simulink model "TrailerSoftware"  (R2019b)
settings: Solver=FixedStepDiscrete  StartTime=0.0  StopTime=inf  FixedStep=update  RelTol=1e-3  EnableMultiTasking=on
values from neighbouring files (symbols this model uses):
  countmax1 = 2500    [ProductionMfile.m]
  countmax2 = 2500    [ProductionMfile.m]
  HeaterIntGain = .0008    (= 0.0008)    [ProductionMfile.m]
  HeatGain = 10    [ProductionMfile.m]
  Intll = 0    [ProductionMfile.m]
  MaxCondPressure = 350    [ProductionMfile.m]
  MinSP = 1    [ProductionMfile.m]
  PostGain100 = 0.0002    [ProductionMfile.m]
  PostGain150 = 0.0005    [ProductionMfile.m]
  PostGain200 = 0.0004    [ProductionMfile.m]
  PostGain300 = 0.0008    [ProductionMfile.m]
  PostInit150 = 12    [ProductionMfile.m]
  PostIntulC = 65    [ProductionMfile.m]
  PostPGain = 0    [ProductionMfile.m]
  PreGain100 = 0.0005    [ProductionMfile.m]
  PreGain150 = 0.0005    [ProductionMfile.m]
  PreGain200 = 0.0003    [ProductionMfile.m]
  PreGain300 = 0.0008    [ProductionMfile.m]
  PreInit150 = 30    [ProductionMfile.m]
  PreIntulC = 65    [ProductionMfile.m]
  PreIntulDH = 65    [ProductionMfile.m]
  PrePGain = 0    [ProductionMfile.m]
  SatPress = [10 20 30 40 50 60 70 80 90 100 110 120 130 140 150 160 170      180 190 200 210 220 230 240 250 260 270 280 290 300 310 320 330      340 350 360 370 380 390 400 410 420 430 440 450 460 470 480 490      500]    [ProductionMfile.m]
  SatTemp = [-29.497 -2.4046 15.401 29.047 40.267 49.88 58.338 65.922 72.819      79.159 85.037 90.526 95.68 100.55 105.16 109.54 113.73 117.73 121.57      125.26 128.82 132.25 135.56 138.77 141.88 144.89 147.82 150.67 153.44      156.15 158.78 161.35 163.85 166.3 168.7 171.04 173.33 175.58 177.77      179.93 182.04 184.11 186.14 188.14 190.09 192.01 193.9 195.75 197.58      199.37]    [ProductionMfile.m]
  SHGain = 2    [ProductionMfile.m]
  SizeCANMatrix = 80    [ProductionMfile.m]
  SizeCOBIDVector = 10    [ProductionMfile.m]
  update = 0.002    [ProductionMfile.m]
undefined symbols (not defined in the file or in its folder): DiscIntNeverNeededParam, PostDGain, PreDGain, Ratio100, Ratio150, Ratio200, Ratio300
libraries: simulink x60, c2837xDlib x35, xpcutilitieslib x24, c2802xlib x8, c280xlib x7, etargetslib x4, svdutilitieslib x2, c2000lib x1
(part 6 of 8)

== matlab function TrailerSoftware/Subsystem/State Machine ==
  data: OutputDiscretes1Out output double size=[16,1]; modeout output; powerselectout output; OpenByPassValve output; DiscreteInput1 input; time input; MBV input; OutputDiscretes2Out output double size=[16,1]; DiscreteInput2 input; MaxPressureout output; ReadATMPress output; CR3 input; CR4 input; FRSettingOut output; stateout output; StartAC output; SuctionPressure input; CurrentStateOut output; StartACDH output; HeaterTempCom output; UseHeater output; CoolTempCom output; BiPassExpanValveCom output; CompressorOnOut output; ResetAC output; CompExitTemp input; warning1 output; warning2 output; warning3 output; fault1 output; fault2 output; fault3 output; debugout output; CR3out output; CR4out output; CompLiquidLevel2High input; MaxCondPressure parameter; CompHeaterTemp input; MinSP parameter; LiquidInjectionOnOut output; DuctTemp input; PressureFB input; Patm input; PreFreezeWarn input; ResetSM output; InitSM output; TempPot input; ByPassValvePos input; FacilityVoltage input; CondenserPressure input; BlowerLevel input; GearBoxLevel input; Latch output; estopout output; Initcomplete1 input; Initcomplete2 input; td input; GearboxTempSwitch input; PrePlusPost input
function [OutputDiscretes1Out,modeout,powerselectout,OpenByPassValve,...
    OutputDiscretes2Out,MaxPressureout,ReadATMPress,FRSettingOut,stateout,...
    StartAC,CurrentStateOut,StartACDH,HeaterTempCom,...
    UseHeater,CoolTempCom,BiPassExpanValveCom,CompressorOnOut,...
    ResetAC,warning1,warning2,warning3,fault1,fault2,fault3,debugout,...
    CR3out,CR4out,LiquidInjectionOnOut,ResetSM,InitSM,Latch,estopout]...
       = fcn(DiscreteInput1,time,MBV,DiscreteInput2,CR3,CR4,...
    SuctionPressure,CompExitTemp,CompLiquidLevel2High,MaxCondPressure,...
    CompHeaterTemp,MinSP,DuctTemp,PressureFB,Patm,PreFreezeWarn,...
    TempPot,ByPassValvePos,FacilityVoltage,...
    CondenserPressure,BlowerLevel,GearBoxLevel,...
    Initcomplete1,Initcomplete2,td,GearboxTempSwitch,PrePlusPost)
persistent  state tmode UseGenerator UseFacility CompressorHeaterOn...
    time1 time2 Motor powerselect ACShutoffOn EngineOn...
    Fault Latch1 Latch3 Latch4 Latch5 Latch6 Latch7 Latch8...
    Latch9 Latch10 Latch11 Latch12 Latch13 time4 nextstate debug oldtmode...   
    FRSetting MaxPressure Fan1On Fan2On FaultLightOn Latch2...
    CurrentState Warning BypassACShutdown DynagenFault Overpressure...
    Latch14 Latch15 LiquidInjectionOn WarningLightOn CompressorOn Idle ...
    Fan1Onlatch Fan1Ontime Fan2Onlatch Fan2Ontime MotorOnlatch ...
    MotorOntime CompressorOnlatch CompressorOntime HGBypass OilOntime ...
    Oillatch LatchMinSP timerMinSP latchComp OverPressureLatch ...
    timeoverpress Latch16 time5 time6 time7 time8 Latch18 OilPumpOn
    
%Only Comments added 2020/01/11
if isempty(Latch1)
    Latch1 = 0;
    Latch2 = 1;
    Latch3 = 0;
    Latch4 = 0;
    Latch5 = 0;
    Latch6 = 0;
    Latch7 = 0;
    Latch8 = 0;
    Latch9 = 0;
    Latch10 = 0;
    Latch11 = 0;
    Latch12 = 0;
    Latch13 = 0;
    Latch14 = 0;
    Latch15 = 0;
    Latch18 = 0;
    time1 = time;
    time2 = time;
    time4 = time;
    state = 0;
    tmode = 0;
    powerselect = 0;
    FRSetting = 0;
    MaxPressure = 1;
    Fault = zeros(41,1);
    CurrentState = 0;
    Warning = zeros(20,1);
    BypassACShutdown = 0;
    DynagenFault = 0;
    nextstate = 0;
    debug = 0;
    oldtmode = 0;
    Overpressure = 2;
    LiquidInjectionOn = 0;
    Motor = 0;
    ACShutoffOn = 0;
    HGBypass = 0;
    UseGenerator = 0;
    UseFacility = 0;
    CompressorHeaterOn = 0;
    EngineOn = 0;
    Fan1On = 0;
    Fan2On = 0;
    FaultLightOn = 0;
    WarningLightOn = 0;
    CompressorOn = 0;
    Idle = 0;
    Fan1Onlatch = 0;
    Fan1Ontime = 0;
    Fan2Onlatch = 0;
    Fan2Ontime = 0;
    MotorOnlatch = 0;
    MotorOntime = 0;
    CompressorOnlatch = 0;
    CompressorOntime = 0;
    OilPumpOn = 0;
    OilOntime = time;
    Oillatch = 0;
    LatchMinSP = 0;
    timerMinSP = 0;
    latchComp = 0;
    OverPressureLatch = 0;
    timeoverpress = 0;
    CompLiquidLevelLatch = 0;
    Latch16 = 0;
    time5 = 0;
    time6 = 0;
    time7 = 0;
    time8 = 0;
end

% Modbus Vector
% MBV(1,1) = SystemStateValue;
% MBV(2,1) = RunningStateValue;
% MBV(3,1) = EventBitMap1ValueA;
% MBV(4,1) = EventBitMap1ValueB;
% MBV(5,1) = EventBitMap2ValueA;
% MBV(6,1) = EventBitMap2ValueB;
% MBV(7,1) = FaultBitMapValueA;
% MBV(8,1) = FaultBitMapValueA;
% MBV(9,1) = WarningBitMapValueA;
% MBV(10,1) = WarningBitMapValueB;
% MBV(11,1) = GenFreqValue;
% MBV(12,1) = GenVoltValueA;
% MBV(13,1) = GenVoltValueB;
% MBV(14,1) = GenVoltValueC;
% MBV(15,1) = GenCurValueA;
% MBV(16,1) = GenCurValueB;
% MBV(17,1) = GenCurValueC;
% MBV(18,1) = EngineTempValue;
% MBV(19,1) = EngineOilPressValue;
% MBV(20,1) = FuelLevelValue;
% MBV(21,1) = BatteryVoltValue;
% MBV(22,1) = EngineRunHoursValue;

% Board 1
% DisIn1
% 1) Transmission Switch #1
% 2) Transmission Switch #2
% 3) Transmission Switch #3
% 4) Transmission Switch #4  (Input 4 No Longer Used, Trans Switch4 is now
%                             Input 16)
% 5) Blower Motor Over Heat
% 6) spare
% 7) Stop
% 8) spare
% 9) System Mode Switch Position 1
% 10) System Mode Switch Position 2
% 11) System Mode Switch Position 3
% 12) System Mode Switch Position 4
% 13)  Blower #2 Temp Switch            Power Mode Switch NO 
% 14) Blower #1 Temp Switch             Power Mode Switch NC
% 15) Reset/Start
% 16) Blower #3 Temp Switch   (Now Transmission Switch 4 2019/11/13)


% Discrete Output 1 - hot gas bypass
% Discrete Output 2 - Compressor #3 valve
% Discrete Output 3 - Compressor liquid injection
% Discrete Output 4 - Warning light
% Discrete Output 5 - Fault light
% Discrete Output 6 - A/C shutoff valve
% Discrete Output 7 - Compressor #4 valve
% Discrete Output 8 - Pre dir 
% Discrete Output 9 - Pre step
% Discrete Output 10 - Post dir
% Discrete Output 11 - Spare
% Discrete Output 12 - Spare
% Discrete Output 13 - Spare
% Discrete Output 14 - Spare
% Discrete Output 15 - Spare
% Discrete Output 16 - Spare
% A/D
% ScaledAtoD1 1 -  
% ScaledAtoD1 2 -  
% ScaledAtoD1 3 -  
% ScaledAtoD1 4 -  
% ScaledAtoD1 5 -  
% ScaledAtoD1 6 -  
% ScaledAtoD1 7 - 
% ScaledAtoD1 8 -  
% CAN A/D


% Board 2
% Discrete Input 1 - Fan 1 current switch
% Discrete Input 2 - Operatetor Shutdown
% Discrete Input 3 - Water pump current switch
% Discrete Input 4 - Fan 2 current switch
% Discrete Input 5 - Estop
% Discrete Input 6 - Oil pump current switch
% Discrete Input 7 - Facility current switch
% Discrete Input 8 - Timer relay
% Discrete Input 9 - Motor current switch
% Discrete Input 10 - Generator current switch
% Discrete Input 11 - spare
% Discrete Input 12 - Compressor 1 current switch
% Discrete Input 13 - spare
% Discrete Input 14 - spare
% Discrete Input 15 - Compressor 2 current switch
% Discrete Input 16 - spare

% Discrete 1 Output - Spare
% Discrete 2 Output - Idle
% Discrete 3 Output - Oil Pump Relay
% Discrete 4 Output - Compressor Contactor 1
% Discrete 5 Output - Compressor Contactor 2
% Discrete 6 Output - Spare
% Discrete 7 Output - Fan1
% Discrete 8 Output - Fan2
% Discrete 9 Output - Genset
% Discrete 10 Output - Facility
% Discrete 11 Output - Spare
% Discrete 12 Output - Engine On/Off
% Discrete 13 Output - Compressor Heater
% Discrete 14 Output - Spare
% Discrete 15 Output - Water Pump
% Discrete 16 Output - Motor
estopout = 0;
Latch = uint32(0);
Latch = bitset(Latch,1,uint8(Latch1));
Latch = bitset(Latch,2,uint8(Latch2));
Latch = bitset(Latch,3,uint8(Latch3));
Latch = bitset(Latch,4,uint8(Latch4));
Latch = bitset(Latch,5,uint8(Latch5));
Latch = bitset(Latch,6,uint8(Latch6));
Latch = bitset(Latch,7,uint8(Latch7));
Latch = bitset(Latch,8,uint8(Latch8));
Latch = bitset(Latch,9,uint8(Latch9));
Latch = bitset(Latch,10,uint8(Latch10));
Latch = bitset(Latch,11,uint8(Latch11));
Latch = bitset(Latch,12,uint8(Latch12));
Latch = bitset(Latch,13,uint8(Latch13));
Latch = bitset(Latch,14,uint8(Latch14));
Latch = bitset(Latch,15,uint8(Latch15));

OutputDiscretes1Out = zeros(16,1);
OutputDiscretes2Out = zeros(16,1);
OpenByPassValve = 0;
MaxPressureout = MaxPressure;
ReadATMPress = 0;
FRSettingOut = FRSetting;
stateout = state;
countwarning = 0;
warning1 = 0;
warning2 = 0;
warning3 = 0;
Reset = DiscreteInput1(15,1);
StartAC = 0;
CurrentStateOut = CurrentState;
StartACDH = 0;
UseHeater = 0;
BiPassExpanValveCom = 0;
CR3BP = CR3;
CR4BP = CR4;
Estop = DiscreteInput2(5); % Estop = 1 OK
if time < 5 
    modeout = 0;
    powerselectout = 0;
    debugout = 0;
    HeaterTempCom = 0;
    CoolTempCom = 0;
    CompressorOnOut = 0;
    ResetAC = 0;
    fault1 = 0;
    fault2 = 0;
    fault3 = 0;
    CR3out = 0;
    CR4out = 0;
    LiquidInjectionOnOut = 0;
    ResetSM = 1;
    InitSM = 0;
    ReadATMPress = 1; 
    return
end
ResetAC = 1;
ResetSM = 0;
InitSM = 0;
if time > 5 && Initcomplete1 == 0 && Initcomplete2 == 0
    InitSM = 1;
end
OvertempVector = zeros(4,1);
if DiscreteInput1(14) == 0  % Blower #1
    OvertempVector(1,1) = 1;
end
if DiscreteInput1(13) == 0 % Blower #2
    OvertempVector(2,1) = 1;
end
% Blower3 temp input now used for transmission switch 4, 2019-11-13
%if DiscreteInput1(16) == 0 % Blower #3
%    OvertempVector(3,1) = 1;
%end 
if GearboxTempSwitch == 0
    OvertempVector(4,1) = 1;
end
SysModePos1 = DiscreteInput1(8);
SysModePos2 = DiscreteInput1(9);
SysModePos3 = DiscreteInput1(6);
SysModePos4 = DiscreteInput1(7);
PowerModeNO = DiscreteInput1(11);
PowerModeNC = DiscreteInput1(10);
Stop = DiscreteInput1(12);
Fan1CurrentSwitch = DiscreteInput2(1);
Fan2CurrentSwitch = DiscreteInput2(4);
OilPumpCurrentSwitch = DiscreteInput2(6);
Timer = DiscreteInput2(8);
MotorIsOn = DiscreteInput2(9);
Compressor1CurrentSwitch = DiscreteInput2(12);
Compressor2CurrentSwitch = DiscreteInput2(15);
MotorNotOverheat = 1;
CompressorShutDown = DiscreteInput2(8,1);
LimitSwitch1 = DiscreteInput1(1);
LimitSwitch2 = DiscreteInput1(2);
LimitSwitch3 = DiscreteInput1(3);
LimitSwitch4 = DiscreteInput1(16);
% Blower3 temp input, DiscreteInput1(16), now used for
% transmission limit switch4, instead of DiscreteInput1(4), 2019-11-13
 BlowerOilFault = 0;
if BlowerLevel >= 1.4
    BlowerOilFault = 1;
end
 GearBoxOilFault = 0;
%if GearBoxLevel >= 1.4
%    GearBoxOilFault = 1;
%end
CompLiquidLevelFault = 0;
if (CompLiquidLevel2High < 1.4) 
    if Latch16 == 0
        time5 = time;
        Latch16 = 1;
    end
    if (time - time5) > 30
        CompLiquidLevelFault = 1;
    end
else
    Latch16 = 0;
end
% Determine the selection of the power switch
if PowerModeNO == 0 && PowerModeNC == 0 % Off
    powerselect = 0; % 
end
if  PowerModeNO == 1 && PowerModeNC == 0
    powerselect = 1; % Generator
end
if PowerModeNO == 1 && PowerModeNC == 1
    powerselect = 2; % Facilility Power
end
% Determine the selction of the mode switch
% Idle = Discrete Input 8 is 1
% De-Hum = Discrete Input 11 is 1
% Cool = Discrete Input 9 is 1
% Heat = Discrete Input 10 is 1
if SysModePos1 == 1
    tmode = 1; % Idle
end
if SysModePos2 == 1
    tmode = 2; % De-Hum
end
if SysModePos3 == 1
    tmode = 3; % Cool
end   
if SysModePos4 == 1
    tmode = 4; % Heat Blower
end 
if Reset == 1 && Latch8 == 1 && Latch10 == 0 % Reset is pushed
    Latch3 = 1;
    oldtmode = tmode;
    Latch10 = 1;
end
% Determine the blower set point
if LimitSwitch1 == 1 && LimitSwitch2 == 0 ... % 100 lbm/min
        && LimitSwitch3 == 0 && LimitSwitch4 == 1  
    FRSetting = 100;
    MaxPressure = 5.75;
    Overpressure = 6.5;
end
if LimitSwitch1 == 1 && LimitSwitch2 == 0 ...  % 150 lbm/min
        && LimitSwitch3 == 1 && LimitSwitch4 == 0 
    FRSetting = 150;
    MaxPressure = 5.75;
    Overpressure = 6.5;
end
if LimitSwitch1 == 0 && LimitSwitch2 == 1 ... % 200 lbm/min
        && LimitSwitch3 == 0 && LimitSwitch4 == 1  
    FRSetting = 200;
    MaxPressure = 3.25;
    Overpressure = 4.25;
end
if LimitSwitch1 == 0 && LimitSwitch2 == 1 ... % 300 lbm/min
        && LimitSwitch3 == 1 && LimitSwitch4 == 0  
    FRSetting = 300;
    MaxPressure = 1.25;
    Overpressure = 3.00;
end 

%Transitions from one mode to another
if Reset == 1 && (CurrentState == 700 || CurrentState == 1300 || ...
        CurrentState == 2300 || CurrentState == 3300 || CurrentState == 4300 ||...
        CurrentState ==5300 || CurrentState == 6300 || ...
        CurrentState == 700 || CurrentState == 700) && tmode ~= oldtmode     
   if powerselect == 1 && tmode == 1 && oldtmode == 3  % Generator from Cool to idle
       BypassACShutdown = 0;
       state = 700;
       time1 = time;
   end
   if powerselect == 1 && tmode == 1 && oldtmode == 2  % Generator from Dehumidifying to idle
       BypassACShutdown = 0;
       state = 700;
       time1 = time;
   end
   if powerselect == 1 && tmode == 1 && oldtmode == 4  % Generator from Blower and Heat to idle
       BypassACShutdown = 1;
       state = 700;
       time1 = time;
   end
   if powerselect == 1 && tmode == 2 && oldtmode == 1  % From Idle to De-Hum
        state = 1100;
        time1 = time;
    end
   if powerselect == 1 && tmode == 3 && oldtmode == 1  % Generator from idle to Cool
       state = 2100;
       time1 = time;
   end
   if powerselect == 1 && tmode == 4 && oldtmode == 1  % Generator from idle to Blower and Heat
       state = 3100;
       time1 = time;
   end
   if powerselect == 1 && tmode == 2 && oldtmode == 3 % Generator and Cool to Generator and Dehumidifying
       state = 1300;
       time1 = time;
   end
   if powerselect == 1 && tmode == 3 && oldtmode == 2  % Generator and Dehumidifying to Generator and Cool
       state = 2100;
       time1 = time;
   end
   if powerselect == 1 && tmode == 4 && oldtmode == 2  % Generator Power and Dehumidifying to Generator Power and Heat
       state = 1400;
       time1 = time;
   end
   if powerselect == 1 && tmode == 4 && oldtmode == 3  % Generator and Cool to Generator Heat
       state = 2400;
       time1 = time;
   end
   if powerselect == 1 && tmode == 3 && oldtmode == 4   % Generator Heat to Generator and Cool
       state = 2220;
       time1 = time;
   end
   if powerselect == 1 && tmode == 2 && oldtmode == 4   % Generator Heat to Generator and Dehumidify
       state = 1220;
       time1 = time;
   end
   if powerselect == 2 && tmode == 2 && oldtmode == 2  % Facilility Power and Cool to Facilility Power and Dehumidifying
       state = 4300;
       time1 = time;
   end
   if powerselect == 2 && tmode == 3 && oldtmode == 2  % Facilility Power and Dehumidifying to Facilility Power and Cool
       state = 5300;
       time1 = time;
   end
   if powerselect == 2 && tmode == 3 && oldtmode == 1  % Facilility Power and Dehumidifying to Facilility Power and Heat
       state = 4400;
       time1 = time;
   end
   if powerselect == 2 && tmode == 4 && oldtmode == 3  % Facilility Power and Cool to Facilility Power Heat
       state = 5400;
       time1 = time;
   end
   if powerselect == 2 && tmode == 3 && oldtmode == 4   % Facilility Power Heat to Facilility Power and Cool
       state = 5220;
       time1 = time;
   end
   if powerselect == 2 && tmode == 2 && oldtmode == 4   % Facilility Power Heat to Facilility Power and Cool
       state = 4220;
       time1 = time;
   end    
   oldtmode = tmode;
end
    
if Latch11 == 0 % Used to set initial configuration
    if tmode == 1 &&  powerselect == 0 && Latch9 == 0 
        Latch8 = 1;  % Latch8 indicates that the powerselect and tmode have been set to 0
        Latch3 = 0;  % Latch3 indicates that the reset button has been pushed
        Latch9 = 1;  % Latch9 prevent this section of code from being repeated
    end
    if Latch3 == 1 && Latch8 == 1 
        Latch3 = 0;
        Latch8 = 0;
        if powerselect == 1 && tmode == 1  % Idle
            state = 500;
            time1 = time;
        end
        if powerselect == 1 && tmode == 2  % De-Hum
            state = 1000;
            time1 = time;
        end
        if powerselect == 1 && tmode == 3  % Generator and Cool
            state = 2000;
            time1 = time;
        end
        if powerselect == 1 && tmode == 4  % Generator, Blower and Heat
            state = 3000;
            time1 = time;
        end
        if powerselect == 2 && tmode == 2  % Facilility, Blower and De-Hum
            state = 4000;
            time1 = time;
        end
        if powerselect == 2 && tmode == 3  % Facilility, Blower and Cool
            state = 5000;
            time1 = time;
        end
        if powerselect == 2 && tmode == 4  % Facilility, Blower and Heat
            state = 6000;
            time1 = time;
        end
        nextstate = state;
        Latch11 = 1;
    end 
end
if (Estop == 0 && (state > 0)) && time > 5 % Estop
    state = 11000;
    CurrentState = 2;
    estopout = 1;
    if CompressorOn == 0
        BypassACShutdown = 1;
    end
end
if BlowerOilFault == 1  % || GearBoxOilFault == 1  
    state = 11000;
    CurrentState = 4;
    if CompressorOn == 0
        BypassACShutdown = 1;
    end
end
if (PressureFB > Overpressure) && (Patm ~= 0) || OverPressureLatch == 1 % Duct over pressure
    if OverPressureLatch == 0
        timeoverpress =  time;
        OverPressureLatch = 1;
    end
    if (time - timeoverpress) > 2
        state = 11000;
        CurrentState = 3;
        Motor = 0; % Super Charger Motor On/Off
        if CompressorOn == 0
            BypassACShutdown = 1;
        end
    end
    if (PressureFB <= Overpressure)
        OverPressureLatch = 0;
    end
end
if OvertempVector(1,1) == 1 % Blower 1 is overheated
    state = 11000;
    CurrentState = 5;
    if CompressorOn == 0
        BypassACShutdown = 1;
    end
end
if OvertempVector(2,1) == 1 % Blower 2 is overheated
    state = 11000;
    CurrentState = 6;
    if CompressorOn == 0
        BypassACShutdown = 1;
    end
end
% Blower3 temp input now used for transmission switch 4, 2019-11-13
%if OvertempVector(3,1) == 1 % Blower 3 is overheated
%    state = 11000;
%    CurrentState = 7;
%    if CompressorOn == 0
%        BypassACShutdown = 1;
%    end
%end
if OvertempVector(4,1) == 1 % Gearbox is overheated
    state = 11000;
    CurrentState = 8;
    if CompressorOn == 0
        BypassACShutdown = 1;
    end
end

if Fan1On == 1 
    if Fan1Onlatch == 0
        Fan1Ontime = time;
        Fan1Onlatch = 1;
    end
%    if ((time - Fan1Ontime) > 10) && Fan1CurrentSwitch ~= 1
%        CurrentState = 10;
%        state = 11000;
%    end
else
    Fan1Onlatch = 0;
end
if Fan2On == 1 
    if Fan2Onlatch == 0
        Fan2Ontime = time;
        Fan2Onlatch = 1;
    end
%    if ((time - Fan2Ontime) > 10) && Fan2CurrentSwitch ~= 1
%        CurrentState = 11;
%        state = 11000;
%    end
else
    Fan2Onlatch = 0;
end
if Motor == 1
    if MotorOnlatch == 0
        MotorOntime = time;
        MotorOnlatch = 1;
    end
%    if ((time - MotorOntime) > 10) && (MotorIsOn ~= 1 ...
%            || OilPumpCurrentSwitch ~= 1)
% if statement below substituted for one above
% because of errant blower motor current sensor port 
% on computer indicated a fault, 4/25/2019
% Sensor was not connected and leads were shorted to 
% fool computer to think current was always present
    %if ((time - MotorOntime) > 10) && OilPumpCurrentSwitch ~= 1
    %    CurrentState = 12;
    %    state = 11000;
    %end
else
    MotorOnlatch = 0;
end
if OilPumpCurrentSwitch ~= 1 && OilPumpOn == 1
    % gearbox oil pump commanded on but no oil pressue
    if Latch18 == 0
        Latch18 = 1;
        time8 = time;
    end
    if time - time8 > 30
        CurrentState = 31;
        BypassACShutdown = 0;
        state = 11000;
    end
else
    Latch18 = 0;
end




CompressorCurSwitchWarning = 0;
if CompressorOn == 1
    if CompressorOnlatch == 0
        CompressorOntime = time;
        CompressorOnlatch = 1;
    end
    if ((time - CompressorOntime) > 10) && ...
            (Compressor1CurrentSwitch ~= 1 ||...
            Compressor2CurrentSwitch ~= 1)
           CompressorCurSwitchWarning = 1;
    end
else
    CompressorOnlatch = 0;
end 
% Dynagen Faults

if (bitget(uint32(MBV(7,1)),6) == 1)  % Low fuel level
    CurrentState = 14;
    state = 11000;
    if CompressorOn == 0
        BypassACShutdown = 1;
    end
end
if (bitget(uint32(MBV(7,1)),9) == 1)  % Low Battery
    CurrentState = 15;
    state = 11000;
    if CompressorOn == 0
        BypassACShutdown = 1;
    end
end
if (state < 4000)  
    if (bitget(uint32(MBV(7,1)),1) == 1)  % Overcrank
        CurrentState = 16;
        state = 11000;
        if CompressorOn == 0
            BypassACShutdown = 1;
        end
    end
    if (bitget(uint32(MBV(7,1)),2) == 1)  % Engine failed to stop
        CurrentState = 17;
        state = 11000;
        if CompressorOn == 0
            BypassACShutdown = 1;
        end
    end
    if (bitget(uint32(MBV(7,1)),4) == 1)  % High engine temperature 
        CurrentState = 18;
        state = 11000;
        if CompressorOn == 0
            BypassACShutdown = 1;
        end
    end
    if (bitget(uint32(MBV(7,1)),5) == 1) && Idle == 0 % Low Oil pressure during rate speed
        CurrentState = 19;
        state = 11000;
        if CompressorOn == 0
            BypassACShutdown = 1;
        end
    end
    if EngineOn == 1
        if Oillatch == 0 && Idle == 1
            Oillatch = 1;
            OilOntime = time;
        end
        if MBV(19,1) < 9 && Idle == 1 && (time - OilOntime) > 20
            CurrentState = 20;
            state = 11000;
            if CompressorOn == 0
                BypassACShutdown = 1;
            end
        end
    else
        Oillatch = 0;
    end
    if (bitget(uint32(MBV(7,1)),7) == 1)  % Under speed
        CurrentState = 21;
        state = 11000;
        if CompressorOn == 0
            BypassACShutdown = 1;
        end
    end
    if (bitget(uint32(MBV(7,1)),8) == 1) % Over speed
        CurrentState = 22;
        state = 11000;
        if CompressorOn == 0
            BypassACShutdown = 1;
        end
    end
    if (bitget(uint32(MBV(7,1)),10) == 1)  % High battery voltage
        CurrentState = 23;
        state = 11000;
        if CompressorOn == 0
            BypassACShutdown = 1;
        end
    end
    if (bitget(uint32(MBV(7,1)),11) == 1)  % Low Coolant level
        CurrentState = 24;
        state = 11000;
        if CompressorOn == 0
            BypassACShutdown = 1;
        end
    end
    if (bitget(uint32(MBV(7,1)),14) == 1)  % Low AC frequency
        CurrentState = 25;
        state = 11000;
        if CompressorOn == 0
            BypassACShutdown = 1;
        end
    end
    if (bitget(uint32(MBV(7,1)),15) == 1)  % High AC frequency
        CurrentState = 26;
        state = 11000;
        if CompressorOn == 0
            BypassACShutdown = 1;
        end
    end
    if (bitget(uint32(MBV(7,1)),16) == 1)  % Low AC voltage
        CurrentState = 27;
        state = 11000;
        if CompressorOn == 0
            BypassACShutdown = 1;
        end
    end
    if (bitget(uint32(MBV(7,1)),17) == 1)  % High AC voltage
        CurrentState = 28;
        state = 11000;
        if CompressorOn == 0
            BypassACShutdown = 1;
        end
    end
end

if Timer == 1 % 24 volts has been shut off
    CurrentState = 29;
    if CompressorOn == 1
        state = 11000;
        BypassACShutdown = 0;
    else
        BypassACShutdown = 1;
    end
end
if Stop == 1  % Operator shutdown
    if CompressorOn == 1
        BypassACShutdown = 0;
    else
        BypassACShutdown = 1;
    end
    state = 11000;
    time1 = time;
    CurrentState = 30;
end

CoolTempCom = min(max(45,abs(TempPot)*(1)+45),140); % 0% = 45 deg F 100% = 140
HeaterTempCom = CoolTempCom;

% Compressor exit overheat
if CompExitTemp > 205 % Turn on liquid injection
    LiquidInjectionOn = 1;
end
if CompExitTemp < 199  % Turn off liquid injection
    LiquidInjectionOn = 0;
end 

if Timer == 1
    CurrentState = 29;
    if CompressorOn == 1
        state = 11000;
        BypassACShutdown = 0;
    else
        BypassACShutdown = 1;
    end
end

switch state
    case 0 % mode and power select is set to off
        OpenByPassValve = 1;
        CurrentState = 0;
        time1 = time;
    case 500
        CurrentState = 500;
        if MBV(1,1) == 150  % Wait Dynagen is in Auto
            OpenByPassValve = 1;           
            EngineOn = 1; % Start/On Engine
            state = 600;
            time1 = time;
        end
    case 600
        CurrentState = 600;
        EngineOn = 1; % Start/On Engine
        Idle = 1;  
    case 700
        OpenByPassValve = 1;
        LiquidInjectionOn = 0; % Turn off liquid injection to the compressor
        CompressorHeaterOn = 0; % Comp Heater on/off.
        if BypassACShutdown == 0 
            % open both expansion valves
            ACShutoffOn = 0; % Turn on/off A/C Shutoff 
            if (time - time1) > 30
                HGBypass = 0; % Hot gas bypass valve is turned off
            end
            BiPassExpanValveCom = 1;
            if (time - time1) > 60 
                 CompressorOn = 0; % Compressor On/Off
                 Latch5 = 1;
                if (time - time1) > 65 
                    Motor = 0; % Super Charger Motor On/Off
                end
            end
            if (time - time1) > 95 
                Fan1On = 0; % Turn off Fan1
            end
            if (time - time1) > 100 
                Fan2On = 0; % Turn off Fan2
                Idle = 1;
            end
            if (time - time1) > 101 
                UseGenerator = 0; % Use Generator On/Off
            end
        else
            ACShutoffOn = 0; % Turn on/off A/C Shutoff
            HGBypass = 0; % Hot gas bypass valve is turned on
            CompressorHeaterOn = 0; % Comp Heater on/off.
            CompressorOn = 0; % Compressor On/Off
            if (time - time1) > 5 
                Motor = 0; % Super Charger Motor On/Off
            end
            if (time - time1) > 20 
                Fan1On = 0; % Turn off Fan1
            end
            if (time - time1) > 25
                Fan2On = 0; % Turn off Fan2
                Idle = 1;
            end
            if (time - time1) > 26
                UseGenerator = 0; % Use Generator On/Off
            end
        end
    case 1000 % Generator and Blower
        CurrentState = 1000;
        OpenByPassValve = 1;  
        if Latch4 == 0 
            Latch4 = 1;
            time1 = 0;
        end 
        if MBV(1,1) == 150  % Wait Dynagen is in Auto        
            state = 1100;
            time1 = time;
        end
        
    case 1100 
        EngineOn = 1; % Start/On Engine
        OilPumpOn = 1; % Turn on geatbox oil pump
        UseGenerator = 1; % Use Generator On/Off
        CurrentState = 1100;
        Idle = 0;  
        OpenByPassValve = 1;
         % By-pass valve is greater than 90% and engine is running and
         % engine temp greater than 120 deg F
        if (ByPassValvePos > 90) && (time - time1) > 30 &&...
                (MBV(1,1) == 156) && (MBV(18,1) > 120) &&...
                (CompLiquidLevelFault == 0) && (MBV(18,1) < 250)
            state = 1200;         
            time1 = time;
            CompressorHeaterOn = 0; % Comp Heater on/off.
        end
        if (time - time1) > 3*60  % Go to
            % shutdown, it took too long to start the engine.
            state = 11000;
            CurrentState = 1101;
            time1 = time;
            BypassACShutdown = 1;
        end
        if powerselect == 0 % Turn Off power
            state = 11000;
            time1 = time;
            CurrentState = 1102;
            BypassACShutdown = 1;
        end
        if CompLiquidLevelFault == 1  % Liquid refrigerant level too high
            CurrentState = 1116;
            if (time - time4) > 7200 
                state =11000;
                BypassACShutdown = 1;
                CurrentState = 1117;
                time1 = time;
                CompressorHeaterOn = 0; % Comp Heater on/off.
            end
            if CompHeaterTemp < 150 
                CompressorHeaterOn = 1; % Comp Heater on/off.
            end
            if CompHeaterTemp > 160 
                CompressorHeaterOn = 0; % Comp Heater on/off.
            end
        else
            time4 = time;
            CompressorHeaterOn = 0; % Comp Heater on/off.
        end
        
    case 1200
        EngineOn = 1; % Start/On Engine     
        OilPumpOn = 1; % Turn on geatbox oil pump
        UseGenerator = 1; % Use Generator On/Off
        OpenByPassValve = 1;
        CurrentState = 1200;
        if time-time1 > 10 
           Motor = 1; % Super Charger Motor On/Off 
           state = 1210;
           time1 = time;
        end        
        if powerselect == 0 % Turn Off power
            state = 11000;
            time1 = time;
            CurrentState = 1202;
            BypassACShutdown = 1;
        end
        
    case 1210
        EngineOn = 1; % Start/On Engine
        OilPumpOn = 1; % Turn on geatbox oil pump
        Motor = 1; % Super Charger Motor On/Off
        UseGenerator = 1; % Use Generator On/Off
        if (time-time1) > 3 
            Fan1On = 1; % Turn on Fan1
        end
        if (time-time1) > 6 
            Fan2On = 1; % Turn on Fan2
        end
        OpenByPassValve = 1;
        CurrentState = 1210;
        if (MotorIsOn == 1) && ((time-time1) > 10)  % Verify motor power is on
            BypassACShutdown = 1;
            state = 1220;
            time1 = time;
        end
        if time-time1 > 10.1  % Motor is not running
            state = 11000;
            time1 = time;
            CurrentState = 1212;
            BypassACShutdown = 1; 
        end  
        if powerselect == 0 % Turn Off power
            state = 11000;
            time1 = time;
            CurrentState = 1213;
            BypassACShutdown = 1;
        end
        if SuctionPressure < MinSP 
            if LatchMinSP == 0
                timerMinSP = time;
                LatchMinSP = 0;
            end
            if (time - timerMinSP) > 60
                CompressorOn = 0; % Compressor On/Off
                state = 11000;
                time1 = time;
                CurrentState = 1214;
                ACShutoffOn = 0; % Turn off A/C Shutoff
                HGBypass = 0; % Hot gas bypass valve is turned off
                BypassACShutdown = 1;
            end
        else
            LatchMinSP = 0;
        end
        if CompLiquidLevelFault == 1 && Latch6 == 0 
             state =11000;
             BypassACShutdown = 1;
             CurrentState = 1217;
        else
            Latch6 = 1;
        end
        if MotorNotOverheat ~= 1  % Blower motor overheated
            CurrentState = 1216;
            state = 11000;
            BypassACShutdown = 1; 
        end
        
    case 1220
        BypassACShutdown = 0;
        EngineOn = 1; % Start/On Engine
        OilPumpOn = 1; % Turn on geatbox oil pump
        Motor = 1; % Super Charger Motor On/Off
        UseGenerator = 1; % Use Generator On/Off
        Fan1On = 1; % Turn on Fan1
        Fan2On = 1; % Turn on Fan2
        CurrentState = 1220;
        if time-time1 > 10 
            state = 1300;
            time1 = time;
        end 
        CR3BP = 1;
        CR4BP = 0;
        ResetAC = 0;
%        ACShutoffOn = 1; % Turn on A/C Shutoff
%        HGBypass = 1; % Hot gas bypass valve is turned on
        StartACDH = 1;
        if powerselect == 0 % Turn Off power
            state = 11000;
            time1 = time;
            CurrentState = 1221;
            BypassACShutdown = 0;
        end
        if SuctionPressure < MinSP 
            if LatchMinSP == 0
                timerMinSP = time;
                LatchMinSP = 0;
            end
            if (time - timerMinSP) > 60
                CompressorOn = 0; % Compressor On/Off
                state = 11000;
                time1 = time;
                CurrentState = 1222;
                ACShutoffOn = 0; % Turn off A/C Shutoff
                HGBypass = 0; % Hot gas bypass valve is turned off
                BypassACShutdown = 0;
            end
        else
            LatchMinSP = 0;
        end
        if CompressorShutDown == 1   % Compressor has stopped
             CompressorOn = 0; % Compressor On/Off
            ACShutoffOn = 0; % Turn off A/C Shutoff
            HGBypass = 0; % Hot gas bypass valve is turned off
            if (time - time4) > 2 
                state = 11000;
                time1 = time;
                CurrentState = 1223; 
                StartAC = 0;
                BypassACShutdown = 0;
            end
        else
            time4 = time;
        end
        if MotorNotOverheat ~= 1  % Blower motor overvheated
            CurrentState = 1225;
            state = 11000;
            BypassACShutdown = 0;
        end
        if CondenserPressure > MaxCondPressure % Maximum Condenser pressure
            CurrentState = 1226;
            state = 11000;
            BypassACShutdown = 0;
        end
%Commented out due to errant blower current sensor input, 4/25/2019        
%        if (MotorIsOn ~= 1) && ((time-time1) > 5)  % SC Over current tripped
%            CurrentState = 1229;
%            state = 11000;
%            BypassACShutdown = 0;
%        end
        time6 = time; 
        
    case 1300 % Wait for shutdown
        CurrentState = 1300;
        EngineOn = 1; % Start/On Engine
        OilPumpOn = 1; % Turn on geatbox oil pump
        UseGenerator = 1; % Use Generator On/Off
        Motor = 1; % Super Charger Motor On/Off
        Fan1On = 1; % Turn on Fan1
        Fan2On = 1; % Turn on Fan2
        StartACDH = 1;
        ResetAC=0;
        if (PrePlusPost < 20) || (latchComp == 1)
                        % CurrentState = 1351;
            if ((time-time6) > 180)
                latchComp = 1;
                        % CurrentState = 1353;
                ACShutoffOn = 0; % Turn off A/C Shutoff 
                HGBypass = 0; % Hot gas bypass valve is turned off
                BiPassExpanValveCom = 1;   % open both expansion valves
                if ((time - time6) > (180+30))  
                    CompressorOn = 0; % Compressor Off
                        % CurrentState = 1355;
                end
            end            
        else
            ACShutoffOn = 1; % Turn On A/C Shutoff
            HGBypass = 1; % Hot gas bypass valve is turned on
            CompressorOn = 1; % Compressor On/Off
            time6 = time; 
                        % CurrentState = 1357;
        end
        UseHeater = 1;
        if DuctTemp > 150  % Check if duct temperature  is too high
            CurrentState = 1310;
            state = 11000;
            time1 = time;  
        end       
        if powerselect == 0 % Turn Off power
            state = 11000;
            time1 = time;
            CurrentState = 1302;
        end
        if SuctionPressure < MinSP 
            if LatchMinSP == 0
                timerMinSP = time;
                LatchMinSP = 0;
            end
            if (time - timerMinSP) > 60
                CompressorOn = 0; % Compressor On/Off
                state = 11000;
                time1 = time;
                CurrentState = 1303;
                ACShutoffOn = 0; % Turn off A/C Shutoff
                HGBypass = 0; % Hot gas bypass valve is turned off
                BypassACShutdown = 0;
            end
        else
            LatchMinSP = 0;
        end
        if CompressorShutDown == 1   % Compressor has stopped
            CompressorOn = 0; % Compressor On/Off
            ACShutoffOn = 0; % Turn off A/C Shutoff
            HGBypass = 0; % Hot gas bypass valve is turned off
            if (time - time4) > 2 
                state = 11000;
                time1 = time;
                CurrentState = 1304; 
                StartAC = 0;
                BypassACShutdown = 1;
            end
        else
            time4 = time;
        end

        if MotorNotOverheat ~= 1  % Blower motor overheated
            CurrentState = 1306;
            state = 11000;
            BypassACShutdown = 1; 
            time1 = time;
        end       
        if CondenserPressure > MaxCondPressure  % Maximum Condenser pressure
            CurrentState = 1307;
            state = 11000;
            BypassACShutdown = 0;
            time1 = time;
        end
        if state ~= 11000 
            if nextstate == 1400 
                state = 1400;
                BypassACShutdown = 0;
                time1 = time;
            end
        end
%Commented out due to errant blower current sensor input, 4/25/2019         
%        if (MotorIsOn ~= 1) && ((time-time1) > 5)  % SC Over current tripped
%            CurrentState = 1308;
%            state = 11000;
%            BypassACShutdown = 1;
%            time1 = time;
%        end
        if CompLiquidLevelFault == 1 || Latch12 == 1 
            Latch12 = 1;
            ACShutoffOn = 0; % Turn on/off A/C Shutoff 
            HGBypass = 0; % Hot gas bypass valve is turned off
            if (time - time2) > 30 
               Latch12 = 0; 
               ACShutoffOn = 1; % Turn on/off A/C Shutoff
               HGBypass = 1; % Hot gas bypass valve is turned on
            end
        else
            time2 = time;
            Latch12 = 0;
        end

%        if PreFreezeWarn == 1 
%            time1 = time;
%            Latch14 = 1;
%            CurrentState = 1321;
%        end

    case 1400 % Transition from cool to heat
        CurrentState = 1400; 
        % open both expansion valves
        ACShutoffOn = 0; % Turn on/off A/C Shutoff 
        if (time - time1) > 30
            HGBypass = 0; % Hot gas bypass valve is turned off
        end
        BiPassExpanValveCom = 1;
        if ((time - time1) > 60) && (BypassACShutdown == 0) || (Latch13 == 1) 
            CompressorOn = 0; % Compressor On/Off
            Latch13 = 1;
            CurrentState = 1401;
            if (time - time1) > 2*60  
                state = 3300;
                Latch13 = 0;
            end
        end
    case 2000 % Generator and Cool
        CurrentState = 2000;
        OpenByPassValve = 1;  
        if Latch4 == 0 
            Latch4 = 1;
            time1 = time;
        end
        if MBV(1,1) == 150  % Is in Auto
            % Command the bypass valve full open
            OpenByPassValve = 1;
            EngineOn = 1; % Start/On Engine       
            state = 2100;
            time1 = time;
            BypassACShutdown = 0;
        end
    case 2100 
        EngineOn = 1; % Start/On Engine
        OilPumpOn = 1; % Turn on geatbox oil pump
        UseGenerator = 1; % Use Generator On/Off
        CompressorHeaterOn = 0; % Comp Heater on/off.
        CurrentState = 2100;
        Idle = 0; 
        OpenByPassValve = 1;
         % By-pass valve is greater than 90% engine temperature is greater
         % than 120 deg F&& MBV(18,1) > 120 and liquid freon is lower than
         % the liquid level,
        if (ByPassValvePos > 90) && (time - time1) > 30 &&...
                (MBV(1,1) == 156) && (MBV(18,1) > 120) && ...
                (MBV(18,1) < 250) && (CompLiquidLevelFault == 0) 
            state = 2200;         
            time1 = time;
            CompressorHeaterOn = 0; % Comp Heater on/off.
        end
        if powerselect == 0 % Turn Off power
            state = 11000;
            time1 = time;
            CurrentState = 2102;
            BypassACShutdown = 1;
        end
        if CompLiquidLevelFault == 1  % % Liquid refrigerant level too high
            CurrentState = 2116;
            if (time - time4) > 7200 
                state =11000;
                BypassACShutdown = 1;
                CurrentState = 2117;
                time1 = time;
                CompressorHeaterOn = 0; % Comp Heater on/off.
            end
            
            if CompHeaterTemp < 150 
                CompressorHeaterOn = 1; % Comp Heater on/off.
            end
            if CompHeaterTemp > 160 
                CompressorHeaterOn = 0; % Comp Heater on/off.
            end
        else
            time4 = time;
            CompressorHeaterOn = 0; % Comp Heater on/off.
        end
    case 2200
        EngineOn = 1; % Start/On Engine   
        OilPumpOn = 1; % Turn on geatbox oil pump
        UseGenerator = 1; % Use Generator On/Off
        OpenByPassValve = 1;
        CurrentState = 2200;
        if time-time1 > 10 
           Motor = 1; % Super Charger Motor On/Off 
           state = 2210;
           time1 = time;
        end
        if powerselect == 0 % Turn Off power
            state = 11000;
            time1 = time;
            CurrentState = 2202;
            BypassACShutdown = 1;
        end    
        if MotorNotOverheat ~= 1  % Blower motor overvheated
            CurrentState = 2204;
            state = 11000;
            BypassACShutdown = 1; 
            time1 = time;
        end
    case 2210
        EngineOn = 1; % Start/On Engine
        OilPumpOn = 1; % Turn on geatbox oil pump
        Motor = 1; % Super Charger Motor On/Off
        UseGenerator = 1; % Use Generator On/Off
        if (time-time1) > 3 
            Fan1On = 1; % Turn on Fan1
        end
        if (time-time1) > 6 
            Fan2On = 1; % Turn on Fan2
        end
        OpenByPassValve = 1;
        CurrentState = 2210;
        if (MotorIsOn == 1) && ((time-time1) > 10)  % Verify 
            %motor power is on and t delta time is geater than 10 seconds
            state = 2220;
            time1 = time; 
        end
        if time-time1 > 10.1  % Motor not running
            state = 11000;
            time1 = time;
            CurrentState = 2212;
            BypassACShutdown = 1; 
        end  
        if powerselect == 0 % Turn Off power
            state = 11000;
            time1 = time;
            CurrentState = 2213;
            BypassACShutdown = 1;
        end
        if SuctionPressure < MinSP
             CompressorOn = 0; % Compressor On/Off
            state = 11000;
            time1 = time;
            CurrentState = 2214;
            ACShutoffOn = 0; % Turn off A/C Shutoff
            HGBypass = 0; % Hot gas bypass valve is turned off
            BypassACShutdown = 1;
        end
        if MotorNotOverheat ~= 1  % Blower motor overvheated
            CurrentState = 2216;
            state = 11000;
            BypassACShutdown = 1; 
            time1 = time;
        end
    case 2220
        BypassACShutdown = 0;
        EngineOn = 1; % Start/On Engine
        OilPumpOn = 1; % Turn on geatbox oil pump
        Motor = 1; % Super Charger Motor On/Off
        UseGenerator = 1; % Use Generator On/Off
        Fan1On = 1; % Turn on Fan1
        Fan2On = 1; % Turn on Fan2
        CurrentState = 2220;
        CR3BP = 1;
        CR4BP = 0;
        if time-time1 > 10 
            state = 2300;
            time1 = time;
        end 
        if time-time1 > 1 
             CompressorOn = 1; % Compressor On/Off
            ResetAC=0;
        end
        ACShutoffOn = 1; % Turn on A/C Shutoff
        HGBypass = 1; % Hot gas bypass valve is turned on
        StartAC = 1;
        if powerselect == 0 % Turn Off power
            state = 11000;
            time1 = time;
            CurrentState = 2222;
            BypassACShutdown = 0;
        end
        if SuctionPressure < MinSP 
            if LatchMinSP == 0
                timerMinSP = time;
                LatchMinSP = 0;
            end
            if (time - timerMinSP) > 60
                CompressorOn = 0; % Compressor On/Off
                state = 11000;
                time1 = time;
                CurrentState = 1223;
                ACShutoffOn = 0; % Turn off A/C Shutoff
                BypassACShutdown = 0;
                HGBypass = 0; % Hot gas bypass valve is turned off
            end
        else
            LatchMinSP = 0;
        end
        if CompressorShutDown == 1   % Compressor has stopped
             CompressorOn = 0; % Compressor On/Off
            ACShutoffOn = 0; % Turn off A/C Shutoff
            HGBypass = 0; % Hot gas bypass valve is turned off
            if (time - time4) > 2 
                state = 11000;
                time1 = time;
                CurrentState = 2224; 
                StartAC = 0;
                BypassACShutdown = 1;
            end
        else
            time4 = time;         
        end
        if MotorNotOverheat ~= 1  % Blower motor overvheated
            CurrentState = 2226;
            state = 11000;
            BypassACShutdown = 1; 
        end
        if CondenserPressure > MaxCondPressure  % Maximum Condenser pressure
            CurrentState = 2227;
            state = 11000;
            BypassACShutdown = 0;
        end
%Commented out due to errant blower current sensor input, 4/25/2019         
%        if (MotorIsOn ~= 1) && ((time-time1) > 5)  % SC Over current tripped
%            CurrentState = 2229;
%            state = 11000;
%            BypassACShutdown = 1;
%        end
    case 2300 % Wait for shutdown
        EngineOn = 1; % Start/On Engine
        OilPumpOn = 1; % Turn on geatbox oil pump
        UseGenerator = 1; % Use Generator On/Off
        Motor = 1; % Super Charger Motor On/Off
        CompressorOn = 1; % Compressor On/Off
        BypassACShutdown = 0;  
        ResetAC=0;
        ACShutoffOn = 1; % Turn On A/C Shutoff 
        HGBypass = 1; % Hot gas bypass valve is turned on
        Fan1On = 1; % Turn on Fan1
        Fan2On = 1; % Turn on Fan2
        CurrentState = 2300;
        StartAC = 1; 
        if powerselect == 0 % Turn Off power
            state = 11000;
            time1 = time;
            CurrentState = 2302;
        end
        if SuctionPressure < MinSP 
            if LatchMinSP == 0
                timerMinSP = time;
                LatchMinSP = 0;
            end
            
            if (time - timerMinSP) > 60
                CompressorOn = 0; % Compressor On/Off
                state = 11000;
                time1 = time;
                CurrentState = 2303;
                ACShutoffOn = 0; % Turn off A/C Shutoff
                BypassACShutdown = 0;
                HGBypass = 0; % Hot gas bypass valve is turned off
            end
        else
            LatchMinSP = 0;
        end
        if CompressorShutDown == 1   % Compressor has stopped
             CompressorOn = 0; % Compressor On/Off
            ACShutoffOn = 0; % Turn off A/C Shutoff
            HGBypass = 0; % Hot gas bypass valve is turned off
            if (time - time4) > 2 
                state = 11000;
                time1 = time;
                CurrentState = 2304; 
                StartAC = 0;
                BypassACShutdown = 0;
            end
        else
            time4 = time;
        end
        if MotorNotOverheat ~= 1  % Blower motor overvheated
            CurrentState = 2306;
            state = 11000;
            BypassACShutdown = 1; 
            time1 = time;
        end
        if CondenserPressure > MaxCondPressure  % Maximum Condenser pressure
            CurrentState = 2307;
            state = 11000;
            time1 = time;
        end
        if state ~= 11000 
            if nextstate == 2400 
                state = 2400;
                time1 = time;
            end
        end
        if CompLiquidLevelFault == 1 || Latch12 == 1 
            Latch12 = 1;
            ACShutoffOn = 0; % Turn on/off A/C Shutoff 
            HGBypass = 0; % Hot gas bypass valve is turned off
            if (SuctionPressure < 35 || (time - time2) > 20) 
               Latch12 = 0; 
               ACShutoffOn = 1; % Turn on/off A/C Shutoff   
               HGBypass = 1; % Hot gas bypass valve is turned on
            end
        else
            time2 = time;
            Latch12 = 0;
        end
%Commented out due to errant blower current sensor input, 4/25/2019         
%        if (MotorIsOn ~= 1) && ((time-time1) > 5) % SC Over current tripped
%            CurrentState = 2309;
%            state = 11000;
%            BypassACShutdown = 1;
%            time1 = time;
%        end
    case 2400 % Transition from cool to heat
        CurrentState = 2400; 
        % open both expansion valves
        ACShutoffOn = 0; % Turn on/off A/C Shutoff   
        BiPassExpanValveCom = 1;
        if (time- time1) > 30
            HGBypass = 0; % Hot gas bypass valve is turned off
        end
        if ((time - time1) > 60) && (BypassACShutdown == 0) || (Latch13 == 1) 
            CompressorOn = 0; % Compressor On/Off
            Latch13 = 1;
            CurrentState = 2401;
            if (time - time1) > 2*60  
                state = 3300;
                Latch13 = 0;
            end
        end      
    case 3000 % Generator and Heat
        CurrentState = 3000;
        OpenByPassValve = 1; 
        if Latch4 == 0 
            Latch4 = 1;
            time1 = 0;
        end
        if  MBV(1,1) == 150  % Wait 1.1 seconds and is in Auto 
            OpenByPassValve = 1;
            % Start engine            
            EngineOn = 1; % Start/On Engine
            if (time - time1) > 10
                state = 3100;
                time1 = time;
            end
        end
    case 3100 
        EngineOn = 1; % Start/On Engine
        OilPumpOn = 1; % Turn on geatbox oil pump
        CurrentState = 3100;
        OpenByPassValve = 1;
        Idle = 0; 
         % By-pass valve is greater than 90%
        if (ByPassValvePos > 90) && (time - time1) > 30 &&...
            (MBV(1,1) == 156) && (MBV(18,1) > 120) && (MBV(18,1) < 250)
            state = 3200;         
            time1 = time;
        end
        if (time - time1) > 3*60  % Engine
            %failed to start or bipass valve not open
            state = 11000;
            CurrentState = 3101;
            time1 = time;
            BypassACShutdown = 1;
        end
        if powerselect == 0 % Turn Off power
            state = 11000;
            time1 = time;
            CurrentState = 3102;
            BypassACShutdown = 1;
        end
    case 3200
        EngineOn = 1; % Start/On Engine       
        OilPumpOn = 1; % Turn on geatbox oil pump
        UseGenerator = 1; % Use Generator On/Off
        OpenByPassValve = 1;
        CurrentState = 3200;
        if time-time1 > 10 
           Motor = 1; % Super Charger Motor On/Off 
           state = 3210;
           time1 = time;
        end
        if powerselect == 0 % Turn Off power
            state = 11000;
            time1 = time;
            CurrentState = 3202;
        end    
    case 3210
        EngineOn = 1; % Start/On Engine
        OilPumpOn = 1; % Turn on geatbox oil pump
        Motor = 1; % Super Charger Motor On/Off
        UseGenerator = 1; % Use Generator On/Off
        OpenByPassValve = 1;
        CurrentState = 3210;
        if (MotorIsOn == 1) && ((time-time1) > 10)  
            % Verify motor power is on and the delta time is geater than 10 seconds
           state = 3300;
           time1 = time;
        end
        if time-time1 > 10.1 % Motor not running
            state = 11000;
            time1 = time;
            CurrentState = 3212;
            BypassACShutdown = 1; 
        end 
        if powerselect == 0 % Turn Off power
            state = 11000;
            time1 = time;
            CurrentState = 3213;
            BypassACShutdown = 1;
        end
        if MotorNotOverheat ~= 1  % Blower motor overvheated
            CurrentState = 3215;
            state = 11000;
            BypassACShutdown = 1; 
            time1 = time;
        end
%Commented out due to errant blower current sensor input, 4/25/2019         
%        if (MotorIsOn ~= 1) && ((time-time1) > 5)  % SC Over current tripped
%            CurrentState = 3219;
%            state = 11000;
%            BypassACShutdown = 1;
%            time1 = time;
%        end
    case 3300
        EngineOn = 1; % Start/On Engine
        OilPumpOn = 1; % Turn on geatbox oil pump
        Motor = 1; % Super Charger Motor On/Off
        UseGenerator = 1; % Use Generator On/Off
        CurrentState = 3300;
        UseHeater = 1;
        if DuctTemp > 150  % Check if duct temperature  is too high
            CurrentState = 3307;
            state = 11000;
            time1 = time;  
            BypassACShutdown = 1; 
        end
        if powerselect == 0 % Turn Off power
            state = 11000;
            time1 = time;
            CurrentState = 3302;
            BypassACShutdown = 1; 
        end
        if DynagenFault == 1 
            CurrentState = 3303;
            state = 11000;
            BypassACShutdown = 1;
            time1 = time;
        end
        if MotorNotOverheat ~= 1  % Blower motor overheated
            CurrentState = 3304;
            state = 11000;
            BypassACShutdown = 1; 
            time1 = time;
        end
%Commented out due to errant blower current sensor input, 4/25/2019        
%        if (MotorIsOn ~= 1) && ((time-time1) > 5)  % SC Over current tripped
%            CurrentState = 3309;
%            state = 11000;
%            BypassACShutdown = 1;
%            time1 = time;
%        end
    case 4000 % Facilility and Blower
        if FacilityVoltage < 300 && (time - time1) > 1 
            CurrentState = 4001; %#ok<NASGU>
            state = 11000;
            time1 = time;
        end
        CurrentState = 4000;
        latchComp = 0;
        OpenByPassValve = 1;  
        if Latch4 == 0 
            Latch4 = 1;
            time1 = 0;
        end 
            
        if (time - time1) > 1.25  % Wait 1.25 sec    
            state = 4100;
            time1 = time;
        end
                
    case 4100 
        UseFacility = 1; % Use Facility On/Off
        OilPumpOn = 1; % Turn on geatbox oil pump
        CurrentState = 4100;
        OpenByPassValve = 1;
        % By-pass valve is greater than 90% 
        if (ByPassValvePos > 90 && (time - time1) > 30) &&...
                CompLiquidLevelFault == 0 
            state = 4200;         
            time1 = time;
            CompressorHeaterOn = 0; % Comp Heater on/off.
        end
        if powerselect == 0 % Turn Off power
            state = 11000;
            time1 = time;
            CurrentState = 4101;
            BypassACShutdown = 1;
        end
        if CompLiquidLevelFault == 1  % % Liquid refrigerant level too high
            CurrentState = 4116;
            if (time - time4) > 7200 
                state =11000;
                BypassACShutdown = 1;
                CurrentState = 4117;
                time1 = time;
                CompressorHeaterOn = 0; % Comp Heater on/off.
            end
            
            if CompHeaterTemp < 150 
                CompressorHeaterOn = 1; % Comp Heater on/off.
            end
            if CompHeaterTemp > 160 
                CompressorHeaterOn = 0; % Comp Heater on/off.
            end            
        else
            time4 = time;
            CompressorHeaterOn = 0; % Comp Heater on/off.
        end
        
    case 4200
        UseFacility = 1; % Use Facility On/Off
        OilPumpOn = 1; % Turn on geatbox oil pump
        OpenByPassValve = 1;
        CurrentState = 4200;
        if time-time1 > 10 
           Motor = 1; % Super Charger Motor On/Off 
           state = 4210;
           time1 = time;
        end
        if powerselect == 0 % Turn Off power
            state = 11000;
            time1 = time;
            CurrentState = 4202;
            BypassACShutdown = 1;
        end
        if MotorNotOverheat ~= 1  % Blower motor overvheated
            CurrentState = 4203;
            state = 11000;
            BypassACShutdown = 1; 
            time1 = time;
        end
        
    case 4210
        Motor = 1; % Super Charger Motor On/Off
        OilPumpOn = 1; % Turn on geatbox oil pump
        UseFacility = 1; % Use Facility On/Off
        if (time-time1) > 3
            Fan1On = 1; % Turn on Fan1
        end
        if (time-time1) > 6 
            Fan2On = 1; % Turn on Fan2
        end
        OpenByPassValve = 1;
        CurrentState = 4210;
        if (MotorIsOn == 1) && ((time-time1) > 10)  % Verify motor
            %power is on and  delta time is geater than 10 seconds
            BypassACShutdown = 1;
            state = 4220;
            time1 = time;
        end
        if time-time1 > 10.1  % Motor not running
            state = 11000;
            time1 = time;
            CurrentState = 4212;
            BypassACShutdown = 1;
        end  
        if powerselect == 0 % Turn Off power
            state = 11000;
            time1 = time;
            CurrentState = 4213;
            BypassACShutdown = 1;
        end
        if CompLiquidLevelFault == 1 && Latch6 == 0 
             state = 11000;
             BypassACShutdown = 1;
             CurrentState = 4214;
             time1 = time;
        else
            Latch6 = 1;
        end
        if MotorNotOverheat ~= 1  % Blower motor overvheated
            CurrentState = 4215;
            state = 11000;
            BypassACShutdown = 1; 
            time1 = time;
        end
        
    case 4220
        BypassACShutdown = 0;
        Motor = 1; % Super Charger Motor On/Off
        OilPumpOn = 1; % Turn on geatbox oil pump
        UseFacility = 1; % Use Facility On/Off
        Fan1On = 1; % Turn on Fan1
        Fan2On = 1; % Turn on Fan2
        CurrentState = 4220;
        if time-time1 > 10   %Keep CR3 on for first 10 sec of compressor operation
            state = 4300;
            time1 = time;
        end  
        CR3BP = 1;
        CR4BP = 0;
        ResetAC = 0;
        StartACDH = 1;
        if powerselect == 0 % Turn Off power
            state = 11000;
            time1 = time;
            CurrentState = 4221;
            BypassACShutdown = 0;
        end
        if SuctionPressure < MinSP 
             CompressorOn = 0; % Compressor On/Off
            state = 11000;
            time1 = time;
            CurrentState = 4222;
            ACShutoffOn = 0; % Turn off A/C Shutoff
            HGBypass = 0; % Hot gas bypass valve is turned off
            BypassACShutdown = 0;
        end
        if CompressorShutDown == 1   % Compressor has stopped
             CompressorOn = 0; % Compressor On/Off
            ACShutoffOn = 0; % Turn off A/C Shutoff
            HGBypass = 0; % Hot gas bypass valve is turned off
            if (time-time4) > 2 
                state = 11000;
                time1 = time;
                CurrentState = 4223; 
                StartAC = 0;
                BypassACShutdown = 1;
            end
        else
            time4 = time;
        end
        if MotorNotOverheat ~= 1  % Blower motor overvheated
            CurrentState = 4225;
            state = 11000;
            BypassACShutdown = 1;
            time1 = time;
        end
        if CondenserPressure > MaxCondPressure  % Maximum Condenser pressure
            CurrentState = 4226;
            state = 11000;
            BypassACShutdown = 0;
            time1 = time;
        end
        if (MotorIsOn ~= 1) && ((time-time1) > 5)  % SC Over current tripped
            CurrentState = 4229;
            state = 11000;
            BypassACShutdown = 1;
            time1 = time;
        end
        
    case 4300 % Wait for shutdown
        UseFacility = 1; % Use Facility On/Off
        Motor = 1; % Super Charger Motor On/Off
        OilPumpOn = 1; % Turn on geatbox oil pump
        if (PrePlusPost > 35) && (latchComp == 0)
            CompressorOn = 1; % Compressor On/Off   
            time6 = time;
            ACShutoffOn = 1; % Turn on A/C Shutoff
            HGBypass = 1; % Hot gas bypass valve is turned on
        else
            if (time-time6) > 3*60
                Latch14 = 1;
                latchComp = 1;
            end
            time1 = time;    
        end
        UseHeater = 1;
        if DuctTemp > 150  % Check if duct temperature  is too high
            CurrentState = 4310; %#ok<NASGU>
            state = 11000;
            time1 = time;  
        end
        Fan1On = 1; % Turn on Fan1
        Fan2On = 1; % Turn on Fan2
        CurrentState = 4300;
        StartACDH = 1;
        if powerselect == 0 % Turn Off power
            state = 11000;
            time1 = time;
            CurrentState = 4302;
        end
        if SuctionPressure < MinSP 
             CompressorOn = 0; % Compressor On/Off
            state = 11000;
            time1 = time;
            CurrentState = 4303;
            ACShutoffOn = 0; % Turn off A/C Shutoff
            HGBypass = 0; % Hot gas bypass valve is turned off
        end
        if CompressorShutDown == 1   % Compressor has stopped
             CompressorOn = 0; % Compressor On/Off
            ACShutoffOn = 0; % Turn off A/C Shutoff
            HGBypass = 0; % Hot gas bypass valve is turned off
            if (time - time4) > 2
                state = 11000;
                time1 = time;
                CurrentState = 4304; 
                StartAC = 0;
                BypassACShutdown = 1;
            end
        else
            time4 = time;
        end
        if MotorNotOverheat ~= 1  % Blower motor overvheated
            CurrentState = 4305;
            state = 11000;
            BypassACShutdown = 1;
            time1 = time;
        end
        if CondenserPressure > MaxCondPressure  % Maximum Condenser pressure
            CurrentState = 4306;
            state = 11000;
            BypassACShutdown = 0;
            time1 = time;
        end
        if state ~= 11000 
            if nextstate == 4400 
                state = 4400;
                BypassACShutdown = 0;
                time1 = time;
            end
        end
        if CompLiquidLevelFault == 1 || Latch12 == 1 
            Latch12 = 1;
            ACShutoffOn = 0; % Turn on/off A/C Shutoff 
            HGBypass = 0; % Hot gas bypass valve is turned off
            if (SuctionPressure < 35 || (time - time2) > 20) 
               Latch12 = 0; 
               ACShutoffOn = 1; % Turn on/off A/C Shutoff  
               HGBypass = 1; % Hot gas bypass valve is turned on
            end
        else
            time2 = time;
            Latch12 = 0;
        end
        if (MotorIsOn ~= 1) && ((time-time1) > 5)  % SC Over current tripped
            CurrentState = 4309;
            state = 11000;
            BypassACShutdown = 1;
            time1 = time;
        end
        
%        if PreFreezeWarn == 1 
%            time1 = time;
%            Latch14 = 1;
%            PreFreezeWarn = 0;    
%            CurrentState = 4321;
%        end
        if Latch14 == 1 
            ACShutoffOn = 0; % Turn on/off A/C Shutoff   
            BiPassExpanValveCom = 1;   % open both expansion valves
            if (time - time1) > 30
                HGBypass = 0; % Hot gas bypass valve is turned off
            end
            if ((time - time1) > 60) || Latch15 == 1 
                CompressorOn = 0; % Compressor On/Off
                ACShutoffOn = 0; % Turn on/off A/C Shutoff 
                HGBypass = 0; % Hot gas bypass valve is turned off
                CurrentState = 4322;
                Latch15 = 1;
            end
        end
        
    case 4400 % Transition from cool to heat
        CurrentState = 4400; 
        % open both expansion valves
        ACShutoffOn = 0; % Turn on/off A/C Shutoff  
        if (time - time1) > 30
            HGBypass = 0; % Hot gas bypass valve is turned off
        end
        BiPassExpanValveCom = 1;
        if ((SuctionPressure < 20 || (time - time1) > 60) && BypassACShutdown == 0) || Latch13 == 1 
             CompressorOn = 0; % Compressor On/Off
            Latch13 = 1;
            CurrentState = 4401;
            if (time - time1) > 2*60  
                state = 6300;
                Latch13 = 0;
            end
        end
    case 5000 % Facility and Cool
        if FacilityVoltage < 300 && (time - time1) > 1 
            CurrentState = 5001; %#ok<NASGU>
            state = 11000;
            time1 = time;
        end
        CurrentState = 5000;
        OpenByPassValve = 1;  
        if (time - time1) > 1.25  % Wait 1.25 sec and is in Auto
            % Command the bypass valve full open
            OpenByPassValve = 1;
            state = 5100;
            time1 = time;
            BypassACShutdown = 0;
        end
    case 5100 
        UseFacility = 1; % Use Facility On/Off
        OilPumpOn = 1; % Turn on geatbox oil pump
        CurrentState = 5100;
        OpenByPassValve = 1;
        % By-pass valve is greater than 90 
        if (ByPassValvePos > 90 && (time - time1) > 30) && ...
             CompLiquidLevelFault == 0
            state = 5200;         
            time1 = time;
            CompressorHeaterOn = 0; % Comp Heater on/off.
        end
        if (time - time1) > 90 % Bi-pass valve is not open
            state = 11000;
            CurrentState = 5101;
            time1 = time;
            BypassACShutdown = 1;
        end
        if powerselect == 0 % Turn Off power
            state = 11000;
            time1 = time;
            CurrentState = 5102;
            BypassACShutdown = 1;
        end
        if CompLiquidLevelFault == 1  % % Liquid refrigerant level too high
            CurrentState = 5116;
            if (time - time4) > 7200 
                state =11000;
                BypassACShutdown = 1;
                CurrentState = 5117;
                time1 = time;
                CompressorHeaterOn = 0; % Comp Heater on/off.
            end
 
            if CompHeaterTemp < 150 
                CompressorHeaterOn = 1; % Comp Heater on/off.
            end
            if CompHeaterTemp > 160 
                CompressorHeaterOn = 0; % Comp Heater on/off.
            end            
        else
            time4 = time;
            CompressorHeaterOn = 0; % Comp Heater on/off.
        end
    case 5200
        UseFacility = 1; % Use Facility On/Off
        OilPumpOn = 1; % Turn on geatbox oil pump
        OpenByPassValve = 1;
        CurrentState = 5200;
        if time-time1 > 10 && CompLiquidLevelFault == 0
           Motor = 1; % Super Charger Motor On/Off 
           state = 5210;
           time1 = time;
        end
        if powerselect == 0 % Turn Off power
            state = 11000;
            time1 = time;
            CurrentState = 5202;
            BypassACShutdown = 1;
        end    
        if MotorNotOverheat ~= 1  % Blower motor overvheated
            CurrentState = 5203;
            state = 11000;
            BypassACShutdown = 1;
            time1 = time;
        end

    case 5210
        Motor = 1; % Super Charger Motor On/Off
        OilPumpOn = 1; % Turn on geatbox oil pump
        UseFacility = 1; % Use Facility On/Off
        OpenByPassValve = 1;
        CurrentState = 5210;
        if (time-time1) > 3 
            Fan1On = 1; % Turn on Fan1
        end
        if (time-time1) > 6 
            Fan2On = 1; % Turn on Fan2
        end
        if (MotorIsOn == 1) && ((time-time1) > 10)  % Verify 
            %motor power is on and delta time is geater than 10 seconds
           state = 5220;
           time1 = time;
        end
        if time-time1 > 10.1   % Motor not running
            state = 11000;
            time1 = time;
            CurrentState = 5212;
            BypassACShutdown = 1;
        end  
        if powerselect == 0 % Turn Off power
            state = 11000;
            time1 = time;
            CurrentState = 5213;
            BypassACShutdown = 1;
        end
        if SuctionPressure < MinSP 
             CompressorOn = 0; % Compressor On/Off
            state = 11000;
            time1 = time;
            CurrentState = 5214;
            ACShutoffOn = 0; % Turn off A/C Shutoff
            HGBypass = 0; % Hot gas bypass valve is turned off
            BypassACShutdown = 1;
        end
        if CompLiquidLevelFault == 1 && Latch6 == 0 
             state =11000;
             BypassACShutdown = 1;
             CurrentState = 5215;
             time1 = time;
        else
            Latch6 = 1;
        end
        if MotorNotOverheat ~= 1  % Blower motor overvheated
            CurrentState = 5216;
            state = 11000;
            BypassACShutdown = 1;
            time1 = time;
        end
        
    case 5220
        BypassACShutdown = 0;
        Motor = 1; % Super Charger Motor On/Off
        OilPumpOn = 1; % Turn on geatbox oil pump
        UseFacility = 1; % Use Facility On/Off
        Fan1On = 1; % Turn on Fan1
        Fan2On = 1; % Turn on Fan2
        if time-time1 > 15 
            state = 5300;
            time1 = time;
        end 
        CurrentState = 5220;
        CR3BP = 1;
        CR4BP = 0;
        if time-time1 > 10 
            state = 5300;
            time1 = time;
        end 
        if time-time1 > 1 
             CompressorOn = 1; % Compressor On/Off
            ResetAC=0;
        end
        ACShutoffOn = 1; % Turn on A/C Shutoff
        HGBypass = 1; % Hot gas bypass valve is turned on
        StartAC = 1;
        if powerselect == 0 % Turn Off power
            state = 11000;
            time1 = time;
            CurrentState = 5221;
            BypassACShutdown = 0;
        end
        if SuctionPressure < MinSP 
             CompressorOn = 0; % Compressor On/Off
            state = 11000;
            time1 = time;
            CurrentState = 5222;
            ACShutoffOn = 0; % Turn off A/C Shutoff
            HGBypass = 0; % Hot gas bypass valve is turned off
            BypassACShutdown = 0;
        end
        if CompressorShutDown == 1   % Compressor has stopped
             CompressorOn = 0; % Compressor On/Off
            ACShutoffOn = 0; % Turn off A/C Shutoff
            HGBypass = 0; % Hot gas bypass valve is turned off
            if (time-time4) > 2  
                state = 11000;
                time1 = time;
                CurrentState = 5223; 
                StartAC = 0;
                BypassACShutdown = 1;
            end
        else
           time4 = time; 
        end
        if MotorNotOverheat ~= 1  % Blower motor overvheated
            CurrentState = 5224;
            state = 11000;
            BypassACShutdown = 1;
            time1 = time;
        end
        if CondenserPressure > MaxCondPressure  % Maximum Condenser pressure
            CurrentState = 5225;
            state = 11000;
            BypassACShutdown = 0;
            time1 = time;
        end
        if (MotorIsOn ~= 1) && ((time-time1) > 5)  % SC Over current tripped
            CurrentState = 5229;
            state = 11000;
            BypassACShutdown = 1;
            time1 = time;
        end
        
    case 5300 % Wait for shutdown
        UseFacility = 1; % Use Facility On/Off
        Motor = 1; % Super Charger Motor On/Off
        OilPumpOn = 1; % Turn on geatbox oil pump
        CompressorOn = 1; % Compressor On/Off
        ACShutoffOn = 1; % Turn On A/C Shutoff 
        HGBypass = 1; % Hot gas bypass valve is turned on
        Fan1On = 1; % Turn on Fan1
        Fan2On = 1; % Turn on Fan2
        if CurrentState ~= 5300 
            ResetAC=0;
        end
        CurrentState = 5300;
        StartAC = 1;
        if powerselect == 0 % Turn Off power
            state = 11000;
            time1 = time;
            CurrentState = 5302;
        end
        if SuctionPressure < MinSP 
             CompressorOn = 0; % Compressor On/Off
            state = 11000;
            time1 = time;
            CurrentState = 5303;
            BypassACShutdown = 1;
            ACShutoffOn = 0; % Turn off A/C Shutoff
            HGBypass = 0; % Hot gas bypass valve is turned off
        end
        if CompressorShutDown == 1   % Compressor has stopped
             CompressorOn = 0; % Compressor On/Off
            ACShutoffOn = 0; % Turn off A/C Shutoff
            HGBypass = 0; % Hot gas bypass valve is turned off
            if (time-time4) > 2 
                state = 11000;
                time1 = time;
                CurrentState = 5304; 
                StartAC = 0;
                BypassACShutdown = 1;
            end        
        else
            time4 = time;
        end
        if MotorNotOverheat ~= 1  % Blower motor overvheated
            CurrentState = 5305;
            state = 11000;
            BypassACShutdown = 1;
            time1 = time;
        end
        if CondenserPressure > MaxCondPressure  % Maximum Condenser pressure
            CurrentState = 5306;
            state = 11000;
            BypassACShutdown = 0;
            time1 = time;
        end
        if state ~= 11000 
            if nextstate == 5400 
                state = 5400;
                BypassACShutdown = 0;
                time1 = time;
            end
        end
        if CompLiquidLevelFault == 1 || Latch12 == 1 
            Latch12 = 1;
            ACShutoffOn = 0; % Turn on/off A/C Shutoff  
            HGBypass = 0; % Hot gas bypass valve is turned off
            if (SuctionPressure < 35 || (time - time2) > 20) 
               Latch12 = 0; 
               HGBypass = 1; % Hot gas bypass valve is turned on
               ACShutoffOn = 1; % Turn on/off A/C Shutoff   
            end
        else
            time2 = time;
            Latch12 = 0;
        end
        if (MotorIsOn ~= 1) && ((time-time1) > 5)  % SC Over current tripped
            CurrentState = 5309;
            state = 11000;
            BypassACShutdown = 1;
            time1 = time;
        end
    case 5400 % Transition from cool to heat
        CurrentState = 5400;
        % open both expansion valves
        ACShutoffOn = 0; % Turn on/off A/C Shutoff   
        BiPassExpanValveCom = 1;
        if (time - time1) > 30
            HGBypass = 0; % Hot gas bypass valve is turned off
        end
        if ((time - time1) > 60) && (BypassACShutdown == 0) || (Latch13 == 1) 
            CompressorOn = 0; % Compressor On/Off
            ACShutoffOn = 0; % Turn on/off A/C Shutoff 
            HGBypass = 0; % Hot gas bypass valve is turned off
            Latch13 = 1;
            CurrentState = 5401;
            if (time - time1) > 2*60  
                state = 6300;
                Latch13 = 0;
            end
        end     
    case 6000 % Facilility and Heat
        if FacilityVoltage < 300 && (time - time1) > 1 
            CurrentState = 6001; %#ok<NASGU>
            state = 11000;
            time1 = time;
        end
        CurrentState = 6000;
        OpenByPassValve = 1;  
        if Latch4 == 0 
            Latch4 = 1;
            time1 = 0;
        end
        if (time - time1) > 1.1  % Wait 
            OpenByPassValve = 1;
            state = 6100;
            time1 = time;
        end
    case 6100 
        CurrentState = 6100;
        OpenByPassValve = 1;
         % By-pass valve is greater than 90%
        if (ByPassValvePos > 90 && (time - time1) > 30) 
            state = 6200;         
            time1 = time;
        end
        if (time - time1) > 90  % Valve is not open
            state = 11000;
            CurrentState = 6101;
            time1 = time;
            BypassACShutdown = 1;
        end
        if powerselect == 0 % Turn Off power
            state = 11000;
            time1 = time;
            CurrentState = 6102;
            BypassACShutdown = 1;
        end
    case 6200 
        UseFacility = 1; % Use Facility On/Off
        OpenByPassValve = 1;
        OilPumpOn = 1; % Turn on geatbox oil pump
        CurrentState = 6200;
        if time-time1 > 10 
           Motor = 1; % Super Charger Motor On/Off 
           state = 6210;
           time1 = time;
        end
        if powerselect == 0 % Turn Off power
            state = 11000;
            time1 = time;
            CurrentState = 6201;
            BypassACShutdown = 1; 
        end    
        if time-time1 > 20 % Motor not running
            state = 11000;
            time1 = time;
            CurrentState = 6202;
            BypassACShutdown = 1; 
        end 
    case 6210
        Motor = 1; % Super Charger Motor On/Off
        OilPumpOn = 1; % Turn on geatbox oil pump
        UseFacility = 1; % Use Facility On/Off
        OpenByPassValve = 1;
        CurrentState = 6210;
        if (MotorIsOn) && ((time-time1) > 10)  
            % Verify motor power is on and t delta time is geater than 10 seconds
           state = 6300;
           time1 = time;
        end
        if time-time1 > 10.1  % Motor not running
            state = 11000;
            time1 = time;
            CurrentState = 6212;
            BypassACShutdown = 1;
        end  
        if powerselect == 0 % Turn Off power
            state = 11000;
            time1 = time;
            CurrentState = 6213;
            BypassACShutdown = 1;
        end
        if MotorNotOverheat ~= 1  % Blower motor overheated
            CurrentState = 6214;
            state = 11000;
            BypassACShutdown = 1;
        end
        if (MotorIsOn ~= 1) && ((time-time1) > 5)  % SC Over current tripped
            CurrentState = 6229;
            state = 11000;
            BypassACShutdown = 1;
        end

    case 6300
        Motor = 1; % Super Charger Motor On/Off
        OilPumpOn = 1; % Turn on geatbox oil pump
        UseFacility = 1; % Use Facility On/Off
        UseHeater = 1;
        if DuctTemp > 150  % Check if duct temperature  is too high
            CurrentState = 6310;
            state = 11000;
            time1 = time;  
        end   
        if powerselect == 0 % Turn Off power
            state = 11000;
            time1 = time;
            CurrentState = 6302;
        end
        if MotorNotOverheat ~= 1  % Blower motor overvheated
            CurrentState = 6303;
            state = 11000;
            BypassACShutdown = 1;
            time1 = time;
        end
        if (MotorIsOn ~= 1) && ((time-time1) > 5)  % SC Over current tripped
            CurrentState = 6309;
            state = 11000;
            BypassACShutdown = 1;
            time1 = time;
        end       
    case 11000 % Turn engine off and Shutdown
        OpenByPassValve = 1;
        LiquidInjectionOn = 0; % Turn off liquid injection to the compressor
        CompressorHeaterOn = 0; % Comp Heater on/off.
        if BypassACShutdown == 0 
            % open both expansion valves
            ACShutoffOn = 0; % Turn on/off A/C Shutoff 
            if (time - time1) > 30
                HGBypass = 0; % Hot gas bypass valve is turned off
            end
            BiPassExpanValveCom = 1;
            if (time - time1) > 60 
                 CompressorOn = 0; % Compressor On/Off
                 Latch5 = 1;
                if (time - time1) > 65 
                    Motor = 0; % Super Charger Motor On/Off
                end
            end
            if (time - time1) > 95 
                Fan1On = 0; % Turn off Fan1
            end
            if (time - time1) > 100 
                Fan2On = 0; % Turn off Fan2
                Idle = 1;
            end
            if (time - time1) > 101 
                UseGenerator = 0; % Use Generator On/Off
            end
            if ((MBV(18,1) < 185) && Latch5 == 1) &&  (time - time1) > 60*3  
                EngineOn = 0; % Start/On Engine 
                OilPumpOn = 0; % Turn off geatbox oil pump
            end
        else
            ACShutoffOn = 0; % Turn on/off A/C Shutoff
            HGBypass = 0; % Hot gas bypass valve is turned on
            CompressorHeaterOn = 0; % Comp Heater on/off.
             CompressorOn = 0; % Compressor On/Off
            if (time - time1) > 5 
                Motor = 0; % Super Charger Motor On/Off
            end
            if (time - time1) > 20 
                Fan1On = 0; % Turn off Fan1
            end
            if (time - time1) > 25
                Fan2On = 0; % Turn off Fan2
                Idle = 1;
            end
            if (time - time1) > 26
                UseGenerator = 0; % Use Generator On/Off
            end
            if (time - time1) > 60*3 
                EngineOn = 0; % Start/On Engine
                OilPumpOn = 0; % Turn off geatbox oil pump
            end
        end
        
        % Faults

        if CurrentState == 1212  || CurrentState == 2212 ||...
                CurrentState == 3212 || CurrentState == 4212  ||...
                CurrentState == 5212 || CurrentState == 6212 % Blower motor is not running
            Fault(1,1) = 101;
        end
        if CurrentState == 1101 || CurrentState == 2101 ||...
                CurrentState == 3101 || CurrentState == 4212 ||...
                CurrentState == 5101 || CurrentState == 6101  % Engine 
            % failed to start or bi-pass valve not open
            Fault(2,1) = 102;
        end
        if CurrentState == 1214 || CurrentState == 1222 ||...
                CurrentState == 1303 || CurrentState == 2214 ||...
                CurrentState == 2223 || CurrentState == 2303 ||...
                CurrentState == 3222 || CurrentState == 4222 ||...
                CurrentState == 4303 ||...|| CurrentState == 5222 ||...
                CurrentState == 5303  % Refrigerant pressure too low
            Fault(3,1) = 103;
        end
        if CurrentState == 1223 || CurrentState == 1304 ||...
             CurrentState == 2224 || CurrentState == 2304 ||...
             CurrentState == 4223 || CurrentState == 4304 ||...
             CurrentState == 5214 || CurrentState == 5223 ||...
             CurrentState == 5304  % Compressor has shut down
            Fault(19,1) = 119;
        end
        if CurrentState == 1306 ||...
                CurrentState == 1216 || CurrentState == 2216 || ...
                CurrentState == 2204 || CurrentState == 2306 ||... 
                CurrentState == 3215 || CurrentState == 3304 ||...
                CurrentState == 4203 || CurrentState == 4225 ||...
                CurrentState == 4305 || CurrentState == 5203 ||...
                CurrentState == 5216 || CurrentState == 5224 ||...
                CurrentState == 5305 || CurrentState == 6214 ||...
                CurrentState == 6303   % Motor overheated
            Fault(20,1) = 120;
        end
        if CurrentState == 2  % Estop tripped
            Fault(21,1) = 121;
            EngineOn = 0; % Start/On Engine
            Fan1On = 0; % Turn on Fan1
            Fan2On = 0; % Turn on Fan2  
            ACShutoffOn = 0; % Turn on/off A/C Shutoff  
            HGBypass = 0; % Hot gas bypass valve is turned off
            CompressorOn = 0; % Compressor On/Off
            Motor = 0; % Super Charger Motor On/Off
            OilPumpOn = 0;
            UseFacility = 0; % Use Facility On/Off
        end
        if CurrentState == 1117 || CurrentState == 2117 ||...                                                                                                                                                                                                                                                                                                                                                                                                                                                                                                                                                               
                CurrentState == 4117 || CurrentState == 5117  % Freon level too high and heating logic timed out
            Fault(22,1) = 122;
        end
        if CurrentState == 1226 || CurrentState == 1307 || CurrentState == 2227 ||...
            CurrentState == 2307 || CurrentState == 4226 ||...
            CurrentState == 4306 || CurrentState == 5225 ||...
            CurrentState == 5306  % Condenser pressure is too high
            Fault(23,1) = 123;
        end
        if CurrentState == 4001 || CurrentState == 5001 || CurrentState == 6001  % Facility power not on.
            Fault(24,1) = 124;
        end
        if CurrentState == 1218 || CurrentState == 1228 || ... % Lost oil pump for gear box
                CurrentState == 1309 || CurrentState == 2217 || ...
                CurrentState == 2228 || CurrentState == 3218 || ...
                CurrentState == 3308 || CurrentState == 4218 || ...
                CurrentState == 4228 || CurrentState == 4308 || ...
                CurrentState == 5218 || CurrentState == 5228 || ...
                CurrentState == 5308 || CurrentState == 6218 || ...
                CurrentState == 6218 
          %      Fault(25,1) = 125;
        end
        if CurrentState == 1229 || CurrentState == 1308 || ... % SC over current trip
                CurrentState == 2229 || CurrentState == 2309 || ...
                CurrentState == 3219 || CurrentState == 3309 || ...
                CurrentState == 4229 || CurrentState == 4309 || ...
                CurrentState == 5229 || CurrentState == 5309 || ...
                CurrentState == 6229 || CurrentState == 6309 
                Fault(26,1) = 126;
        end
        if CurrentState == 1310 || CurrentState == 3307 || ... % Duct Over-temperature
                CurrentState == 4310 || CurrentState == 6310 
                Fault(27,1) = 127;
        end
        if CurrentState == 3  %Duct Overpressure
                Fault(28,1) = 128;
        end
        if CurrentState == 31  % Loss gear box oil
           Fault(29,1) = 129; 
        end
        if CurrentState == 5  %Blower #1 overheat
          Fault(31,1) = 131;
        end 
        if CurrentState == 6  %Blower #2 overheat
          Fault(32,1) = 132;
        end 
        if CurrentState == 7  %Blower #3 overheat
          Fault(33,1) = 133;
        end 
        if CurrentState == 8  %Gearbox overheat
            Fault(34,1) = 134;
        end
        if CompLiquidLevelFault == 1 % Oil too high
            Fault(35,1) = 135;
        end
        if CurrentState == 10 % No current in Fan1 
            Fault(36,1) = 136;
        end
        if CurrentState == 11 % No current in Fan2  
            Fault(37,1) = 137;
        end
        if CurrentState == 12 % No current in Motor contactor
            Fault(38,1) = 138;
        end
        if CurrentState == 13 % No Current in Compressor contactors
            Fault(39,1) = 139;
        end
   case 20000

end

% Dynagen Faults

if CurrentState == 14  % Low fuel level
    Fault(8,1) = 108;
end
if CurrentState == 15 % Low Battery
    Fault(11,1) = 111;
end
if (CurrentState < 4000 && state == 11000)  
    if CurrentState == 16  % Overcrank
        Fault(4,1) = 104;
    end
    if CurrentState == 17   % Engine failed to stop
        Fault(5,1) = 105;
    end
    if CurrentState == 18  % High engine temperature 
        Fault(6,1) = 106;
    end
    if CurrentState == 19 || CurrentState == 20   % Low Oilpressure
        Fault(7,1) = 107;
    end
    if CurrentState == 21   % Under speed
        Fault(9,1) = 109;
    end
    if CurrentState == 22  % Over speed
        Fault(10,1) = 110;
    end
    if CurrentState == 23   % High battery voltage
        Fault(12,1) = 112;
    end
    if CurrentState == 24  % Low Coolant level
        Fault(13,1) = 113;
    end
    if CurrentState == 25   % Low AC frequency
        Fault(14,1) = 114;
    end
    if CurrentState == 26   % High AC frequency
        Fault(15,1) = 115;
    end
    if CurrentState == 27   % Low AC voltage
        Fault(16,1) = 116;
    end
    if CurrentState == 28  % High AC voltage
        Fault(17,1) = 117;
    end
%    if (bitget(uint32(MBV(7,1)),18) == 1)  % Loss of ECM Comm
%        Fault(18,1) = 118;
%    end
else 
    for i = 4:7 
        Fault(i,1) = 0;
    end
    Fault(9,1) = 0;
    Fault(10,1) = 0;
    for i = 12:18 
        Fault(i,1) = 0;
    end
end
% Warning
Warning = zeros(20,1);
WarningLightOn = 0;
if CurrentState == 1116|| CurrentState == 1117 || CurrentState == 2116 ||...                                                                                                                                                                                                                                                                                                                                                                                                                                                                                                                                                               
    CurrentState == 2117 ||CurrentState == 4116 || CurrentState == 4117 ||...
    CurrentState == 5116 || CurrentState == 5117   
    Warning(17,1) = 217;  % Freon level too high compressor heater on
end
if CurrentState == 1401 || CurrentState == 2401 || ...
        CurrentState == 4401 || CurrentState == 5401 
        Warning(16,1) = 216; % Waiting for compressor pressures to equalize 
end
if (bitget(uint32(MBV(9,1)),8) == 1)  % High Battery Voltage
    Warning(8,1) = 208;
end
if (bitget(uint32(MBV(9,1)),9) == 1)  % Low Battery Voltage
    Warning(9,1) = 209;
end
if (bitget(uint32(MBV(9,1)),6) == 1)  % Low Fuel Level
    Warning(7,1) = 207;
end
if (LimitSwitch1 == 1 && LimitSwitch2 == 0 ... % 100 lbm/min
                && LimitSwitch3 == 0 && LimitSwitch4 == 1) ...
                || (LimitSwitch1 == 1 && LimitSwitch2 == 0 ...  % 150 lbm/min
                && LimitSwitch3 == 1 && LimitSwitch4 == 0) ... 
                || (LimitSwitch1 == 0 && LimitSwitch2 == 1 ... % 200 lbm/min
                && LimitSwitch3 == 0 && LimitSwitch4 == 1) ... 
                || (LimitSwitch1 == 0 && LimitSwitch2 == 1 ... % 300 lbm/min
                && LimitSwitch3 == 1 && LimitSwitch4 == 0)  
else
    Warning(15,1) = 215; % Gear box is in neutral
end

%if PreFreezeWarn == 1
%    Warning(18,1) = 218; % Pre-Cooler is freezing, Bypass Valve Opened
%end

if state < 4000 
    if MBV(1,1) ~= 150 && MBV(1,1) ~= 156  % Engine controller not in Auto
        Warning(2,1) = 202;
    end
    if (bitget(uint32(MBV(9,1)),1) == 1)  % Low engine temperature
        Warning(1,1) = 201;
    end
    if (bitget(uint32(MBV(9,1)),2) == 1)  % High engine temperature
        Warning(3,1) = 203;
    end
    if (bitget(uint32(MBV(9,1)),3) == 1 && Idle ~= 1) ||...
            (Idle == 1 && MBV(19,1) < 13) % Low Oil pressure
        Warning(4,1) = 204;
    end
    if (bitget(uint32(MBV(9,1)),4) == 1)  % Under speed
        Warning(5,1) = 205;
    end
    if (bitget(uint32(MBV(9,1)),5) == 1)  % Over Speed
        Warning(6,1) = 206;
    end
    if (bitget(uint32(MBV(9,1)),11) == 1)  % Over AC frequency
        Warning(11,1) = 211;
    end
    if (bitget(uint32(MBV(9,1)),12) == 1)  % AC under voltage
        Warning(12,1) = 212;
    end
    if (bitget(uint32(MBV(9,1)),13) == 1)  % AC over voltage
        Warning(13,1) = 213;
    end
    if (bitget(uint32(MBV(9,1)),15) == 1)  % AC over current
        Warning(14,1) = 214;
    end 
    if latchComp == 1 % RH too low
         Warning(19,1) = 219;
    end
    if CompressorCurSwitchWarning == 1 % No current to compressor
        Warning(20,1) = 220;
    end
end
    
for i = 1:20
    if Warning(i,1) ~= 0 
%        WarningLightOn = 1; % Turnon Warning light
        countwarning = countwarning + 1;
        if countwarning == 1
            warning1 = Warning(i,1); 
        end
        if countwarning == 2 
            warning2 = Warning(i,1); 
        end
        if countwarning == 3 
            warning3 = Warning(i,1); 
        end 
    end
end
for i = 2:20
    if Warning(i,1) ~= 0
        WarningLightOn = 1; % Turnon Warning light
    end
end
countfault = 0;
fault1 = 0;
fault2 = 0;
fault3 = 0;
for i = 1:41
    if Fault(i,1) ~= 0 
        FaultLightOn = 1; % Turnon Fault light
        countfault = countfault + 1;
        if countfault == 1 
            fault1 = Fault(i,1); 
        end
        if countfault == 2 
            fault2 = Fault(i,1); 
        end
        if countfault == 3 
            fault3 = Fault(i,1); 
        end  
    end
end

CompressorOnOut = 0;
if  CompressorOn == 1 
    CompressorOnOut = 1;
end
LiquidInjectionOnOut = LiquidInjectionOn;
if CompressorOn == 0  % Compressor On/Off
    CR3BP = 0;
    CR4BP = 0;
end
CR3out = CR3BP;
CR4out = CR4BP;
OutputDiscretes1Out(1) = HGBypass;
OutputDiscretes1Out(2) = CR3out;
OutputDiscretes1Out(3) = LiquidInjectionOn;
OutputDiscretes1Out(6) = ACShutoffOn;
OutputDiscretes1Out(7) = CR4out;
OutputDiscretes1Out(8) = FaultLightOn;
OutputDiscretes1Out(4) = WarningLightOn;
modeout = tmode;
powerselectout = powerselect;
debug = double(MBV(2,1));
debugout = debug;
OutputDiscretes2Out(2) = Idle;
OutputDiscretes2Out(3) = OilPumpOn;
OutputDiscretes2Out(4) = CompressorOn;
OutputDiscretes2Out(7) = Fan1On;
OutputDiscretes2Out(8) = Fan2On;
OutputDiscretes2Out(9) = UseGenerator;
OutputDiscretes2Out(10) = UseFacility;
OutputDiscretes2Out(12) = EngineOn;
OutputDiscretes2Out(13) = CompressorHeaterOn;
OutputDiscretes2Out(15) = 1;
OutputDiscretes2Out(16) = Motor;
return
